simulink library "carnot"  (R2013b)
settings: Solver=ode45  StartTime=0.0  StopTime=10.0  RelTol=1e-3
undefined symbols (not defined in the file or in its folder): A, acol, Ahabit, Awin, Azimuth_Angle, AziWin, B, C, c1, c4, capc, caph, CarnotCallbacks_Density, CarnotCallbacks_Enthalpy, CarnotCallbacks_Enthalpy2Temperature, CarnotCallbacks_Entropy, CarnotCallbacks_Evaporation_Enthalpy, CarnotCallbacks_GlobalMessageLevel, CarnotCallbacks_Grashof, CarnotCallbacks_Heat_Capacity, CarnotCallbacks_Kinematic_Viscosity, CarnotCallbacks_Prandtl, CarnotCallbacks_Saturation_Property, CarnotCallbacks_Saturation_Temperature, CarnotCallbacks_Saturation_Value_Water, CarnotCallbacks_Specific_Volume, CarnotCallbacks_Thermal_Conductivity, CarnotCallbacks_Vapour_Content, CarnotCallbacks_Vapour_Pressure, con, cond, d, Dd, density, dfin, dia, DiameterLastPiece, DPConstant, dpipe, DPLinear, DPQuadratic, emission_out, fluid, FluidMix, FluidType, FPC, frame, g, GeodeticHeight, Gwin, heat_capacity, hgt, HP, Hroom, ID, inlet, K, l, lin, lpipe ... (+29)
undefined symbols (not defined in the file): c2, c3, c5, c6, cwall, dactive, height, mc, mID, rho, tau, UAneighbour, UAwall, uloss
libraries: carnot x333, simulink x25, simulink_extras x7
(part 1 of 16)
settings Model: Creator=awohlfei  LastModifiedBy=awohlfei

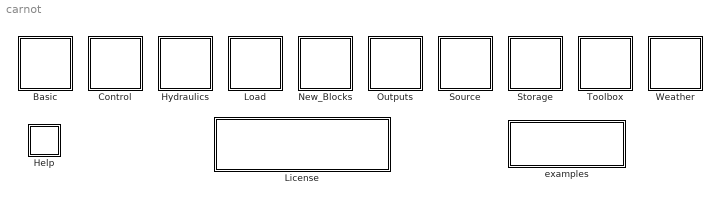
== system carnot ==
  Basic : Subsystem
      mask Display: plot(0,0,100,100,[10,10,40,40,10],[10,40,40,10,10],[50,70,90,50],[30,65,30,30],[20,10,10,20,30,40,40,30,20],[50,60,70,80,80,70,60,50,50])
  Control : Subsystem
      mask Display: plot(0,0,100,100,[70,100,40,10,70,70,10,10],[50,80,80,50,50,20,20,50],[100,70],[50,20],[20,50,50,20,20],[40,40,30,30,40],[62,62,62,61,59,58,58,60],[42,41,39,38,38,40,42,43],[61,62,62,61,60,59,58,58,58,59],[32,31,30,28,27,28,28,30,31,32])
  Help : Subsystem
      settings: OpenFcn=manual
      mask Display: disp('?');
  Hydraulics : Subsystem
      mask Display: plot(0,0,100,100,[15,18,18,15,40,40,46,55,60,60,55,46,40,40,15,10,10,15],[60,53,46,40,40,20,24,24,20,80,85,85,80,60,60,53,46,40],[60,55,46,40],[20,15,15,20])
  License : Subsystem
      mask Display: disp('Carnot 6.0\nfor MATLAB R2013b\nCopyright Solar-Institute Juelich');
  Load : Subsystem
      mask Display: plot(0,0,100,100,[10,20,30,10,30,30,10,10],[30,50,30,30,30,10,10,30],[30,20,10,30,30,10,10],[80,100,80,80,60,60,80],[77,76,70,50],[70,76,80,80],[74,66],[90,90],[70,70],[80,89],[77,76,70,50],[20,26,30,30],[74,66],[40,40],[70,70],[30,39])
  New_Blocks : Subsystem
      mask Display: plot(0,0,100,100,[80,20],[10,10],[70,55,45,30],[10,90,90,10])
  Outputs : Subsystem
      mask Display: plot(0,0,100,100,[90,10,10],[10,10,90],[90,80,70,60,50,10],[65,63,50,26,20,20],[90,70,57,46,40,31,40,50,60,70,90],[78,78,72,60,36,20,20,33,60,70,70],[90,60,45,31,24,21,14,21,30,34,44,59,90],[87,87,85,75,58,35,20,20,37,58,77,83,83])
  Source : Subsystem
      mask Display: plot(0,0,100,100,[30,40,60,70,70,30,30],[50,44,44,50,10,10,50],[50,50],[44,57],[50,46,44,46,50,54,56,54,50],[93,85,70,54,48,54,70,85,93])
  Storage : Subsystem
      mask Display: plot(10,10,90,100,[40,40,45,55,60,60,55,45,40],[84,36,30,30,36,84,90,90,84],[40,35],[77,77],[64,60],[77,77],[40,35],[42,42],[64,60],[42,42])
  Toolbox : Subsystem
      mask Display: plot(0,0,100,100,[10,40,50,40,10,10],[90,90,80,70,70,90],[28,28,22,22],[70,10,10,70],[70,80,80,70,70],[50,50,10,10,50],[77,77],[10,50],[73,73],[10,50],[76,76,74,74],[50,90,90,50])
  Weather : Subsystem
      mask Display: plot(7,7,95,100,[10,7,10,20,30,23,25,40,54,56,50,60,70,73,70,60,20,10],[15,24,34,40,35,42,50,55,50,42,35,40,34,24,15,10,10,15],[70,60,60,70,80,90,90,80,70],[90,80,70,60,60,70,80,90,90],[75,75],[91,97],[75,75],[52,58],[58,52],[75,75],[98,91],[75,75],[63,58],[63,57],[92,86],[92,87],[63,58],[85,92],[92,86],[57,64])
  examples : Subsystem
      settings: OpenFcn=|
      | filepath = '\public\tutorial\examples';
      | oldpath = pwd;
      | cd(fullfile(path_carnot('root'),filepath));
      | [filename, pathname, filterindex] = ...
      | uigetfile( { '*.mdl', ...
      | 'house examples'; ...
      | '*.mdl','MAT-files (*.mat)'; ...
      | '*.*',  'All Files (*.*)'},  'Pick an example');
      | if (filterindex > 0)
      |    open_system(fullfile(pathname,filename));
      | end
      | cd(oldpath);
      mask Display: disp('double click \nto load examples');

== system carnot/Basic ==
  Hydraulics : Subsystem
      mask Display: plot(0,0,100,100,[15,18,18,15,40,40,46,55,60,60,55,46,40,40,15,10,10,15],[60,53,46,40,40,20,24,24,20,80,85,85,80,60,60,53,46,40],[60,55,46,40],[20,15,15,20])
  Material_Properties : Subsystem
      mask Display: plot(10,10,80,80,[30,25,20,25,30,30,40,40,25,10,10,20,20],[60,59,60,61,60,50,32,30,27,30,32,50,60],[50,54,54,50,60,68,70,60,50,45,40,40,44,50],[60,64,70,72,70,67,70,75,77,77,73,65,60,60],[70,65,60,65,70,70,67,64,60],[50,51,50,48,50,15,10,10,15],[60,60],[15,50])
  Pressure_Drop : Subsystem
      mask Display: plot(0,0,100,100,[10,10,40,40,10],[10,40,40,10,10],[50,70,90,50],[30,65,30,30],[20,10,10,20,30,40,40,30,20],[50,60,70,80,80,70,60,50,50])
  Thermal_Models : Subsystem
      mask Display: plot(0,0,100,100,[10,10,40,40,10],[10,40,40,10,10],[50,70,90,50],[30,65,30,30],[20,10,10,20,30,40,40,30,20],[50,60,70,80,80,70,60,50,50])
  Ventilation : Subsystem
      mask Display: plot(0,0,100,100,[10,10,40,40,10],[10,40,40,10,10],[50,70,90,50],[30,65,30,30],[20,10,10,20,30,40,40,30,20],[50,60,70,80,80,70,60,50,50])
  Weather_and_Sun : Subsystem
      mask Display: plot(7,7,95,100,[10,7,10,20,30,23,25,40,54,56,50,60,70,73,70,60,20,10],[15,24,34,40,35,42,50,55,50,42,35,40,34,24,15,10,10,15],[70,60,60,70,80,90,90,80,70],[90,80,70,60,60,70,80,90,90],[75,75],[91,97],[75,75],[52,58],[58,52],[75,75],[98,91],[75,75],[63,58],[63,57],[92,86],[92,87],[63,58],[85,92],[92,86],[57,64])

== system carnot/Control ==
  Controller_Bang_Bang : Subsystem  mask(bang bang controler){deltaTon=5, deltaToff=1, Tmax=95}
      mask prompts: deltaTon "deltaT-on [K]"; deltaToff "deltaT-off [K]"; Tmax "maximum temperature [degree centigrade]"
      mask help:
      | Hysteresis controller for thermal systems. Output is set to zero if Thot or Tcold is bigger than Tmax.
      | deltaT = Thot - Tcold
      mask Help: web(fullfile(path_carnot('help'),'Controller_Bang_Bang.html'),'-helpbrowser')
      mask Display: plot(-30,0,150,100,[70,100,40,10,70,70,10,10],[50,80,80,50,50,20,20,50],[100,70],[50,20],[20,50,50,20,20],[40,40,30,30,40],[62,62,62,61,59,58,58,60],[42,41,39,38,38,40,42,43],[61,62,62,61,60,59,58,58,58,59],[32,31,30,28,27,28,28,30,31,32])
  EnergyMeter : Subsystem  mask(energy meter){}
      mask help: Calculates the power and energy of a fluid flow between inlet and outlet of components.
      mask Help: web(fullfile(path_carnot('help'),'EnergyMeter.html'),'-helpbrowser')
  EnergyMeter_HC : Subsystem  mask(energy meter Heating/Cooling){}
      mask help:
      | Calculates the power and energy of a fluid flow between inlet and outlet of components.
      | Positive power is integrated to the heating energy, negative power is integrated to the cooling energy.
      mask Help: eval('htmlhelp (''chap_4_2e.htm#energy_meter'')');
  Massflow_Sensor : Subsystem  mask(temperature measurement sensor){tc=10, t0=0}
      mask prompts: tc "time constant of sensor [s]"; t0 "initial value [kg/s]"
      mask help: Measurement sensor for temperatures with first-oder hold. Temperature is in degree centigrade.
      mask init:
      | tc = 1/max(tc, 0.001);
      mask Help: web(fullfile(path_carnot('help'),'Massflow_Sensor.html'),'-helpbrowser')
  Max_Run_Time : Subsystem  mask(Maximum Running Time){tmaxrun=5}
      mask prompts: tmaxrun "Maximum operation time in s"
      mask help: Keeps the output to the input level until either the maximum running time is reached or the input is set to zero.
      mask Help: web(fullfile(path_carnot('help'),'Max_Run_Time.html'),'-helpbrowser')
      mask Display:
      | plot(-20,-30,120,100,[10,20,40,60,80,90,90,80,60,40,20,10,10],[40,20,10,10,20,40,60,80,90,90,80,60,40],[55,46],[95,95],[50,50],[90,95],[50,50,24],[88,50,66],[10,13],[50,50],[90,87],[50,50],[50,50],[10,15])
      | disp('\n\nMax On')
  Min_Run_Time : Subsystem  mask(Minimum Running Time){tminrun=2, mv=2}
      mask prompts: tminrun "Minimum operation time in s"; mv "Minimum output value"
      mask help: Once started, the output is kept to the maximum of the input value and the mimimum output for at least the minimum running time.
      mask Help: web(fullfile(path_carnot('help'),'Min_Run_Time.html'),'-helpbrowser')
      mask Display:
      | plot(-20,-30,120,100,[10,20,40,60,80,90,90,80,60,40,20,10,10],[40,20,10,10,20,40,60,80,90,90,80,60,40],[55,46],[95,95],[50,50],[90,95],[50,50,24],[88,50,66],[10,13],[50,50],[90,87],[50,50],[50,50],[10,15])
      | disp('\n\nMin On')
  Min_Stop_Time : Subsystem  mask(Minimum Stop Time){tminstop=15}
      mask prompts: tminstop "Minimum stop time in s"
      mask help: Once stopped, the output is held to zero for at least the minimum stop time.
      mask Help: web(fullfile(path_carnot('help'),'Min_Stop_Time.html'),'-helpbrowser')
      mask Display:
      | plot(-20,-30,120,100,[10,20,40,60,80,90,90,80,60,40,20,10,10],[40,20,10,10,20,40,60,80,90,90,80,60,40],[55,46],[95,95],[50,50],[90,95],[50,50,24],[88,50,66],[10,13],[50,50],[90,87],[50,50],[50,50],[10,15])
      | disp('\n\nMin Off')
  OnOff_switch : Constant  Value=0
      settings: OpenFcn=set_param(gcb,'value',num2str(1-str2num(get_param(gcb,'value'))))
  PowerMeter : Subsystem  mask(power meter){}
      mask help:
      | Calculates the power of a fluid flow between inlet and outlet of components characterized by the THB.
      | Qdot = mdot * cp(Tmean) * (Tout - Tin)
      | Tmean = (Tin+Tout)/2
      mask Help: web(fullfile(path_carnot('help'),'PowerMeter.html'),'-helpbrowser')
  Solar_Radiation_Sensor : Subsystem  mask(measure solar radiation){rad=diffuse, rad_typ=normal to the beam radiation}
      mask prompts: rad "measured radiation"; rad_typ "orientation of the sensor"
      mask help:
      | Extracts the solar radiation in W/m² from the weather data vector.
      |
      | WARNING:
      | For old weather data vectors, their is only one type of tsolar radiation.
      mask init:
      | if (rad_typ == 1)
      |     if (rad == 1)
      |         vector = [3];
      |     elseif (rad == 2)
      |         vector = [4];
      |     else
      |         vector = [3 4];
      |     end
      | else
      |     if (rad == 1)
      |         vector = [16];
      |     elseif (rad == 2)
      |         vector = [17];
      |     else
      |         vector = [16 17];
      |     end
      | end
      mask Help: web(fullfile(path_carnot('help'),'Solar_Radiation_Sensor.html'),'-helpbrowser')
      mask TypeOptions rad: direct | diffuse | global
      mask TypeOptions rad_typ: normal to the beam radiation | fixed (horizontal or inclined)
  Start_Delay : Subsystem  mask(Start Delay){tstartdelay=5}
      mask prompts: tstartdelay "Start delay time in s"
      mask help: The output is delayed for the delay time, than it equal to the input.
      mask Help: web(fullfile(path_carnot('help'),'Start_Delay.html'),'-helpbrowser')
      mask Display:
      | plot(-20,-30,120,100,[10,20,40,60,80,90,90,80,60,40,20,10,10],[40,20,10,10,20,40,60,80,90,90,80,60,40],[55,46],[95,95],[50,50],[90,95],[50,50,24],[88,50,66],[10,13],[50,50],[90,87],[50,50],[50,50],[10,15])
      | disp('\n\nDelay On')
  T_Sensor : Subsystem  mask(temperature measurement sensor){tc=10, t0=20}
      mask prompts: tc "time constant of sensor [s]"; t0 "initial temperature [degree centigrade]"
      mask help: Measurement sensor for temperatures with first-oder hold. Temperature is in degree centigrade.
      mask init:
      | tc = 1/max(tc, 0.001);
      mask Help: web(fullfile(path_carnot('help'),'T_Sensor.html'),'-helpbrowser')
      mask Display: plot(0,0,100,100,[50,55,65,70,70,65,55,45,35,30,30,35,44,50,50],[50,50,60,70,80,90,100,100,90,80,70,60,50,50,-0],[60,40],[90,90],[50,50],[57,90])
  T_Sensor_Surface : Subsystem  mask(surface temperature sensor){pos=[0.1 0.4 0.5 0.9], tdel=1, t0=20}
      mask prompts: pos "relative position 0..1 (0 = bottom, 1 = top)"; tdel "delay-time in s"; t0 "initial temperature in degree centigrade"
      mask help:
      | Surface temperature sensor for a storage. The block breaks the algebraic loop when connecting the node temperature directly to the controller.
      | The relative position can be a vector for several sensors, for example [0.1 0.5 0.9]
      mask init:
      | tdel = max(tdel,0.01);
      | pos = max(0, min(pos, 1));
      mask Help: web(fullfile(path_carnot('help'),'T_Sensor_Surface.html'),'-helpbrowser')
      mask Display: plot(-10,0,110,100,[50,55,65,70,70,65,55,45,35,30,30,35,44,50,50],[50,50,60,70,80,90,100,100,90,80,70,60,50,50,-0],[60,40],[90,90],[50,50],[57,90])
  Window_Control : Subsystem  mask(Window Control){}
      mask help: Control for free driven passive cooling realized by tilted windows.
      mask Help: web(fullfile(path_carnot('help'),'Window_Control.html'),'-helpbrowser')

== system carnot/Help ==

== system carnot/Hydraulics ==
  Flow_Diverter : Subsystem  mask(flow diverter, fixed rate){}
      mask help:
      | The block diverts an incoming massflow according to:
      | mdot1 = mdot * fdiv
      | mdot2 = mdot * (1-fdiv)
      | fdiv is limited to the range [0..1]
      mask Help: web(fullfile(path_carnot('help'),'Flow_Diverter.html'),'-helpbrowser')
      mask Display: plot(0,-5,120,65,[20 45 20 20],[20 30 40 20],[45 70 70 45],[30 20 40 30],[45 35 55 45],[30 10 10 30])
  Flow_Mixer : Subsystem  mask(flow mixer){t=10}
      mask prompts: t "time constant of mixer"
      mask help: Mixes two massflows. The new temperature is calculated by an energy balance. The output f_div may be fed back to the corresponding flow diverter upwards in flowdirection.
      mask init:
      | if t < 0.0001
      |     t = 0.0001;
      |     disp('warning in Flow Mixer: Time constant set to 0.0001')
      | end
      mask Help: web(fullfile(path_carnot('help'),'Flow_Mixer.html'),'-helpbrowser')
      mask Display: plot(-25,-5,95,65,[20 45 20 20],[20 30 40 20],[45 70 70 45],[30 20 40 30],[45 35 55 45],[30 10 10 30])
  Flow_Mixer_Thermostatic : Subsystem  mask(thermostatic flow mixer){t=10}
      mask prompts: t "time constant for valve [s]"
      mask help:
      | The thermostatic flow mixer mixes cold and hot fluid to set a desired temperature and calculates the pressure drop.
      | Use together with flow_diverter_fixed_rate.
      mask init:
      | if t < 0.01
      |     t = 0.01;
      |     disp('Flow mixer thermostatic: time constant set to minimum value 0.01')
      | end
      | t1 = 1/t;
      mask Help: web(fullfile(path_carnot('help'),'Flow_Mixer.html'),'-helpbrowser')
      mask Display: plot(10,0,100,100,[40,60,60,40,40],[60,40,60,40,60],[44,50,56,44],[66,50,66,66],[50,50],[30,50],[56,44],[25,25],[50,50],[10,25])
  Pipe : Subsystem  mask(pipe){dia=0.02, len=10, hgt=5, uloss=100/20/10, cond=0, cwall=1000, t0=20, lin=100/0.2, qua=100/0.2^2, nodes=10}
      mask prompts: dia "diameter [m]"; len "length of pipe [m]"; hgt "static height [m], positive for outlet above"; uloss "heat losses per length [W/(m*K)]"; cond "effective conductivity in axial direction [W/(m*K)]"; cwall "capacity of pipewall per length in [J/(m*K)]"; t0 "initial temperature [degree Celsius]"; lin "pressure drop linear in massflow [Pa*s/kg]"; qua "pressure drop quadratic in massflow [Pa*s²/kg²]"; nodes "number of nodes"
      mask help:
      | Multinode pipe with capacity and simlified pressure drop calculation. The pressure drop is a quadratic function of the massflow. The dependance of the quadratic term on the Reynolds number is neglected. The flow is calculated by the upwind scheme heat conduction between nodes by central differences (Patankar 1980).
      | heat loss: ul = 2*Conductivity*pi*d_in*Length/Length/(d_in*ln(d_out/d_in))
      | The pressure change due to static height can usually be neglected for closes loop pumped systems.
      mask init:
      | if dia < 0.001
      |     dia = 0.001;
      |     disp('Warning in Pipe: diameter set to minimum value 0.001 m')
      | end
      | if len < 0.001
      |     len = 0.001;
      |     disp('Warning in Pipe: length set to minimum value 0.001 m')
      | end
      | if cwall < 0.001
      |     cwall = 0.001;
      |     disp('Warning in Pipe: heat capacity of the wall set to minimum value 0.001 m')
      | end
      | if nodes < 1
      |     nodes = 1;
      |     disp('Warning in Pipe: number of nodes set to minimum 1')
      | end
      mask Help: web(fullfile(path_carnot('help'),'Pipe.html'),'-helpbrowser')
      mask Display: plot(0,0,100,100,[24,27,27,24,75,80,80,75,24,20,20,24],[60,53,46,40,40,46,55,60,60,53,46,40])
  Pipe_Geometry : Subsystem  mask(Pipe Geometry){dia=0.02, len=10, hgt=10, uloss=100/20/10, cond=0, cwall=1000, t0=20, rough=0.04*1e-3, nbend=4, nodes=1}
      mask prompts: dia "diameter [m]"; len "length of pipe [m]"; hgt "static height [m], (positive for outlet above inlet)"; uloss "heat loss per length of pipe [W/(m*K)]"; cond "effective conductivity in the pipe [W/(m*K)]"; cwall "capacity of pipewall per length [J/(m*K)]"; t0 "initial temperature [degree centigrade]"; rough "roughness of pipe [m]"; nbend "number of 90° bends (45° = 0.667)"; nodes "number of nodes"
      mask help:
      | Multinode pipe with capacity and theoretical pressure drop calculation. The flow is calculated by the upwind scheme heat conduction between nodes by central differences (Patankar 1980).
      | heat loss: ul = 2*Conductivity*pi*d_in*Length/Length/(d_in*ln(d_out/d_in))
      | The pressure change due to static height can usually be neglected for closes loop pumped systems.
      mask init:
      | if dia < 0.001
      |     dia = 0.001;
      |     disp('Warning in Pipe: diameter set to minimum value 0.001 m')
      | end
      | if len < 0.001
      |     len = 0.001;
      |     disp('Warning in Pipe: length set to minimum value 0.001 m')
      | end
      | if cwall < 0.001
      |     cwall = 0.001;
      |     disp('Warning in Pipe: heat capacity of the wall set to minimum value 0.001 m')
      | end
      | if nodes < 1
      |     nodes = 1;
      |     disp('Warning in Pipe: number of nodes set to minimum 1')
      | end
      | if nbend < 0
      |     nbend = 0;
      |     disp('Warning in Pipe: number of bends set to minimum 0')
      | end
      | if rough < 0
      |     rough = 0;
      |     disp('Warning in Pipe: roughness of nodes set to minimum 0 m')
      | end
      mask Help: web(fullfile(path_carnot('help'),'Pipe_Geometry.html'),'-helpbrowser')
      mask Display: plot(0,0,90,100,[8,12,16,16,12,8,8],[46,38,46,55,62,55,46],[12,33,48,52,70,73,73,70,50,35,30,12],[38,49,30,30,50,55,65,70,50,70,70,62])
  Pipe_Isolation : Subsystem  mask(pipe with relative isolation thickness){dia=0.02, len=10, hgt=0, isolat=43.72, condiso=0.05, cond=0, cwall=1000, t0=20, lin=100/0.2, qua=100/0.2^2, nodes=10}
      mask prompts: dia "Diameter [m]"; len "Length of pipe [m]"; hgt "difference in static height [m], positive for outlet above"; isolat "Isolation thickness in % (100%: isolation thickness = diameter, minimum 1%)"; condiso "Thermal conductivity of isolation [W/(m*K)]"; cond "Effective conductivity in the pipe [W/(m*K)]"; cwall "capacity of pipewall per length in [J/(m*K)]"; t0 "initial temperature [degree centigrade]"; lin "pressure drop linear in massflow [Pa*s/kg]"; qua "pressure drop quadratic in massflow [Pa*s²/kg²]"; nodes "number of nodes"
      mask help:
      | Multinode pipe with capacity and easy pressure drop calculation. The pressure drop is a quadratic function of the massflow. The dependance of the quadratic term on the Reynolds number is neglected. The flow is calculated by the upwind scheme heat conduction between nodes by central differences (Patankar 1980).
      | Isolation thickness in percent of the diameter. Heat loss:
      | ul = 2*conductivity*pi*d*Length/Length/(d*log(((2*percent+1)d)/d))
      | The pressure change due to static height can usually be neglected for closes loop pumped systems.
      mask init:
      | if dia < 0.001
      |     dia = 0.001;
      |     disp('Warning in Pipe: diameter set to minimum value 0.001 m')
      | end
      | if len < 0.001
      |     len = 0.001;
      |     disp('Warning in Pipe: length set to minimum value 0.001 m')
      | end
      | if cwall < 0.001
      |     cwall = 0.001;
      |     disp('Warning in Pipe: heat capacity of the wall set to minimum value 0.001 m')
      | end
      | if nodes < 1
      |     nodes = 1;
      |     disp('Warning in Pipe: number of nodes set to minimum 1')
      | end
      | if isolat < 1
      |     isolat = 1;
      |     disp('Warning in Pipe: Isolation set to minimum 1%')
      | end
      | uloss = 2*condiso*pi/(log(0.01*isolat*2+1));
      mask Help: web(fullfile(path_carnot('help'),'Pipe_Isolation.html'),'-helpbrowser')
      mask Display: plot(-20,10,130,90,[0,2,5,7,5,2,0],[55,50,50,55,60,60,55],[96,99,100,99,96],[50,50,55,60,60],[10,13,17,19,19,17,13,10],[50,45,45,50,60,65,65,60],[5,15,17,17,15,5],[50,50,52,58,60,60],[17,93,96,96,92,17],[45,45,46,62,65,65])
  Pump_Additional : Subsystem  mask(additional pump){a0=2.0e4, a1=-7000, a2=0 %-3e-3, dia=0.025, t1=5, ua=0, mcp=0, tamb=0}
      mask prompts: a0 "pump characteristic: constant coefficient [Pa]"; a1 "pump characteristic: linear coefficient [Pa*s/kg]"; a2 "pump characteristic: quadratic coefficient [Pa*(s/kg)²]"; dia "diameter at in- and outlet [m]"; t1 "time constant in s"; ua "losses to ambient  in W/K"; mcp "thermal capacity in J/K"; tamb "ambient temperatature in °C"
      mask help: This pump is an additional pump in a circuit. Every circuit must have exactly ONE 'pump_main'. It may have several 'pump_additional' blocks.
      mask init:
      | t=1;
      mask Help: web(fullfile(path_carnot('help'),'Pump_Main.html'),'-helpbrowser')
      mask Display:
      | plot(0,0,100,100,[40,70,40,30,30,40,60,70,70,60,40],[70,50,30,40,60,70,70,60,40,30,30])
      | port_label('input',1,'THB')
      | port_label('input',2,'ctr')
      | port_label('output',1,'THB')
      | port_label('output',2,'Pel')
  Pump_Const : Subsystem  mask(constant pump){mdotmax=1200/3600, dia=0.0157, power=30, p0=3e5, fluid_id=Water, mix=0, UA=3, mcp=4000, tamb=20}
      mask prompts: mdotmax "massflow rate [kg/s]"; dia "diameter at in- and outlet [m]"; power "electric power consumption [W]"; p0 "system pressure in Pa"; fluid_id "fluid"; mix "percentage of fluid mix [0..1]"; UA "losses to ambient in W/K"; mcp "thermal capacity in J/K"; tamb "ambient temperatature in °C"
      mask help:
      | Set constant massflow rate according to the control signal.
      | The pump has a thermal capacity and losses to ambient.
      mask Help: web(fullfile(path_carnot('help'),'Pump_Const.html'),'-helpbrowser')
      mask TypeOptions fluid_id: Water | Air | Cotton Oil | Silicone Oil | Water-Glycol Mix | Tyfocor LS | Water (Constant 20°C) | Air (dry+ constant 20°C)
      mask Display:
      | plot(0,0,100,100,[40,70,40,30,30,40,60,70,70,60,40],[70,50,30,40,60,70,70,60,40,30,30])
      | port_label('input',1,'THB')
      | port_label('input',2,'ctr')
      | port_label('output',1,'THB')
      | port_label('output',2,'Pel')
  Pump_Main : Subsystem  mask(main pump){a0=2.7e4, a1=-1.2e4, a2=-3e-3, dia=0.025, t1=5, p0=3e5, IDchk=off, fluid_id=Water, mix=0, ua=1, mcp=500, tamb=20}
      mask prompts: a0 "constant coefficient a0 [Pa]"; a1 "linear coefficient a1 [Pa*s/kg]"; a2 "quadratic coefficient a2 [Pa*(s/kg)²]"; dia "diameter at in- and outlet [m]"; t1 "time constant in s"; p0 "system pressure in Pa"; IDchk "calculate static pressure in system"; fluid_id "fluid"; mix "percentage of fluid mix [0..1]"; ua "losses to ambient  in W/K"; mcp "thermal capacity in J/K"; tamb "ambient temperatature in °C"
      mask help:
      | This is the main pump in a circuit. Every circuit must have exactly ONE 'Pump_Main'. Use the 'pump_additional' blocks if you want to use more pumps.
      | Calculate massflow by solving the equations:
      |     pressure_drop = c + l*mdot + q*(mdot)²
      |     pump_pressure = a0 + a1*mdot +a2*(mdot)²
      |     with: pressure_drop = pump_pressure
      | The system pressure specified as parameter is the pressure at the outlet of the pump. All pressure drops in the circuit will reduce this pressure.
      mask init:
      | ID = IDchk*10000+10001;
      mask Help: web(fullfile(path_carnot('help'),'Pump_Main.html'),'-helpbrowser')
      mask TypeOptions fluid_id: Water | Air | Cotton Oil | Silicone Oil | Water-Glycol Mix | Tyfocor LS | Water (Constant 20°C) | Air (dry+ constant 20°C)
      mask Display:
      | plot(0,0,100,100,[40,70,40,30,30,40,60,70,70,60,40],[70,50,30,40,60,70,70,60,40,30,30])
      | port_label('input',1,'THB')
      | port_label('input',2,'ctr')
      | port_label('output',1,'THB')
      | port_label('output',2,'Pel')
  Pump_Simple : Subsystem  mask(simple Pump){mdotmax=1200/3600, dia=0.0157, power=30, fluid_id=Water, mix=0, p0=3e5}
      mask prompts: mdotmax "massflow rate [kg/s]"; dia "diameter at in- and outlet [m]"; power "electric power consumption [W]"; fluid_id "fluid"; mix "percentage of fluid mix [0..1]"; p0 "system pressure [Pa]"
      mask help:
      | Set constant massflow rate according to the control signal.
      | The pump is a very basic model, sometimes creating algebraic loops. If you have problems with algebraic loops, use "Pump_const" instead.
      mask Help: web(fullfile(path_carnot('help'),'Pump_Const.html'),'-helpbrowser')
      mask TypeOptions fluid_id: Water | Air | Cotton Oil | Silicone Oil | Water-Glycol Mix | Tyfocor LS | Water (Constant 20°C) | Air (dry+ constant 20°C)
      mask Display:
      | plot(0,0,100,100,[40,70,40,30,30,40,60,70,70,60,40],[70,50,30,40,60,70,70,60,40,30,30])
      | port_label('input',1,'THB')
      | port_label('input',2,'ctr')
      | port_label('output',1,'THB')
      | port_label('output',2,'Pel')
  Thermosyphon : Subsystem  mask(thermosyphon){dia=0.025, fluid_id=water, mix=0, p0=2e5, t1=5}
      mask prompts: dia "diameter at in- and outlet [m]"; fluid_id "fluid"; mix "percentage of fluid mix [0..1]"; p0 "system pressure in [Pa]"; t1 "time constant in s"
      mask help:
      | This block is a model of a "thermosyphon pump". Place it in natural convection systems as you would place a pump.
      | Assure that the sum of heights is zero. Otherwise the simulation will not start.
      | You may check the sum of heights by verifying the "Geodetic Height" in the THB at the inport of this block.
      | If the sum is not zero, the difference is displayed in the subsystem "Stop Simulation".
      mask Help: web(fullfile(path_carnot('help'),'Thermosyphon.html'),'-helpbrowser')
      mask TypeOptions fluid_id: water | air | cotton oil | silicone oil | water-glycol mix | Tyfocor LS
      mask Display:
      | plot(0,0,100,100,[90,10],[80,90],[90,10],[70,80],[90,10],[20,10],[90,10],[30,20],[40,60,40,40],[60,50,40,60])
      | port_label('input',1,'THB')
      | port_label('output',1,'THB')
  Valve : Subsystem  mask(valve){pos_values=[0 0.1 1], dp_values=[1e6 1e6 1]}
      mask prompts: pos_values "position (vector with values 0..1)"; dp_values "QUA : quadratic pressure drop (vector)"
      mask help:
      | The block calculates the pressure drop at a valve. The characteristic is defined by a lookup table for QUA:
      | dp = QUA * mdot^2
      mask Help: web(fullfile(path_carnot('help'),'Valve.html'),'-helpbrowser')
      mask Display: plot(-15,0,115,100,[30,70,70,30,30],[60,40,60,40,60],[60,40],[80,80],[50,50],[50,80])
  Valve_ThermoTset : Subsystem  mask(thermostatic valve){p=3, op=0.5, bl=10, ts=30, dia=0.02, vpos=[0 0.1 1], vqua=[1e6 1e6 1]}
      mask prompts: p "proportional Range [K]"; op "operating point [0..1] (valve position at set temperature)"; bl "play hysteresis []"; ts "first-order hold ts [s]"; dia "diameter [m]"; vpos "Valve position vector [0..1]"; vqua "Vector with quadratic pressure drop in massflow in Pa*s²/kg²"
      mask help:
      | Thermostatic valve for a radiator.
      | set temperature and slope
      | valve position = -slope * (T(sensor) - Toffset)
      mask init:
      | % p=1/p;
      | % op = min(1, max(0, op));
      | % tu = max(tu,0);
      | % ts = max(ts,0);
      | % dia = max(dia, 0.001);
      | %
      mask Help: web(fullfile(path_carnot('help'),'Valve_Thermostatic.html'),'-helpbrowser')
      mask Display:
      | plot(-30,-10,130,110,[20,80,80,20,20],[60,30,60,30,60],[50,50],[45,70],[60,40],[96,96],[50,50],[75,96])
      | port_label('input',1,'THB')
      | port_label('input',2,'Troom')
      | port_label('input',3,'Tset')
      | port_label('output',1,'THB')
  Valve_ThermoTset_fn : Subsystem  mask(thermostatic valve with Kv function){p=3, op=0.5, bl=0.1, ts=30, dia=0.02, kv=0.6, kvs=0.8}
      mask prompts: p "proportional Range [K]"; op "operating point [0..1] (valve position at set temperature)"; bl "play hysteresis [K]"; ts "first-order hold ts [s]"; dia "diameter [m]"; kv "kv value"; kvs "kvs value"
      mask help:
      | Thermostatic valve for a radiator.
      | set temperature and slope
      | valve position = -slope * (T(sensor) - Toffset)
      mask Help: web(fullfile(path_carnot('help'),'Valve_Thermostatic.html'),'-helpbrowser')
      mask Display:
      | plot(-30,-10,130,110,[20,80,80,20,20],[60,30,60,30,60],[50,50],[45,70],[60,40],[96,96],[50,50],[75,96])
      | % port_label('input',1,'THB')
      | % port_label('input',2,'Troom')
      | % port_label('input',3,'Tset')
      | % port_label('output',1,'THB')
  Valve_Thermostatic : Subsystem  mask(thermostatic valve){Tset=20, prange=3, op=0.5, bl=0.1, ts=30, dia=0.02, vpos=[0 0.1 1], vqua=[1e6 1e6 1]}
      mask prompts: Tset "set temperature [degree centigrade]"; prange "proportional Range [K]"; op "operating point [0..1] (valve position at set temperature)"; bl "play hysterersis in K"; ts "first-order hold ts [s]"; dia "diameter [m]"; vpos "Valve position vector [0..1]"; vqua "Vector with quadratic pressure drop in massflow in Pa*s²/kg²"
      mask help:
      | Thermostatic valve for a radiator.
      | set temperature and slope
      | valve position = -slope * (T(sensor) - Toffset)
      mask Help: web(fullfile(path_carnot('help'),'Valve_Thermostatic.html'),'-helpbrowser')
      mask Display:
      | plot(-20,-10,130,110,[20,80,80,20,20],[60,30,60,30,60],[50,50],[45,70],[60,40],[96,96],[50,50],[75,96])
      | port_label('input',1,'THB')
      | port_label('input',2,'Troom')
      | port_label('output',1,'THB')
  Valve_fn : Subsystem  mask(valve with Kv function){kv=0.7, kvs=0.9, op=0.5}
      mask prompts: kv "Kv value"; kvs "Kvs value"; op "Operation point [0..1]"
      mask help:
      | The block calculates the pressure drop at a valve. The characteristic is defined the function:
      | QUA = 2.8e6*(kv/(kvs*(2/(1+exp(-2/op*u(1)))-1)))^2
      | dp = QUA * mdot^2
      mask Help: web(fullfile(path_carnot('help'),'Valve_fn.html'),'-helpbrowser')
      mask Display: plot(-15,0,115,100,[30,70,70,30,30],[60,40,60,40,60],[60,40],[80,80],[50,50],[50,80])

== system carnot/License ==
  note: This file is part of the CARNOT Blockset.
      | 	Copyright (c) 1998-2015, Solar-Institute Juelich of the FH Aachen.
      | 	Additional Copyright for file and models see list auf authors.
      | 	All rights reserved.
      | 	Redistribution and use in source and binary forms, with or without
      | 	modification, are permitted provided that the following conditions are met:
      | 	1. Redistributions of source code must retain the above copyright notice,
      | 	   this list of conditions and the following disclaimer.
      | 	2. Redistributions in binary form must reproduce the above copyright
      | 	   notice, this list of conditions and the following disclaimer in the
      | 	   documentation and/or other materials provided with the distribution.
      | 	3. Neither the name of the copyright holder nor the names of its
      |
      |    contributors may be used to endorse or promote products derived from
      |    this software without specific prior written permission.
      | THIS SOFTWARE IS PROVIDED BY THE COPYRIGHT HOLDERS AND CONTRIBUTORS "AS IS"
      | 	AND ANY EXPRESS OR IMPLIED WARRANTIES, INCLUDING, BUT NOT LIMITED TO, THE
      | 	IMPLIED WARRANTIES OF MERCHANTABILITY AND FITNESS FOR A PARTICULAR PURPOSE
      | 	ARE DISCLAIMED. IN NO EVENT SHALL THE COPYRIGHT HOLDER OR CONTRIBUTORS BE
      | 	LIABLE FOR ANY DIRECT, INDIRECT, INCIDENTAL, SPECIAL, EXEMPLARY, OR
      | 	CONSEQUENTIAL DAMAGES (INCLUDING, BUT NOT LIMITED TO, PROCUREMENT OF
      | 	SUBSTITUTE GOODS OR SERVICES; LOSS OF USE, DATA, OR PROFITS; OR BUSINESS
      | 	INTERRUPTION) HOWEVER CAUSED AND ON ANY THEORY OF LIABILITY, WHETHER IN
      | 	CONTRACT, STRICT LIABILITY, OR TORT (INCLUDING NEGLIGENCE OR OTHERWISE)
      | 	ARISING IN ANY WAY OUT OF THE USE OF THIS SOFTWARE, EVEN IF ADVISED OF
      | 	THE POSSIBILITY OF SUCH DAMAGE.

== system carnot/Load ==
  General : Subsystem
      mask Display: plot(0,0,100,100,[100,0,0],[-0,-0,100],[100,95,81,72,62,54,51,36,26,20,17,15,13,10,0],[10,46,32,57,96,96,31,39,5,1,87,33,47,50,10])
  Hot_Water_Tapping : Subsystem
      mask Display: plot(0,0,100,100,[44,67,67,45,45,40,40,44],[80,80,72,72,60,60,76,80],[60,45],[90,90],[53,53],[80,90],[24,29,70,75,24],[30,10,10,30,30],[42,42],[32,58],[46,44],[34,54],[38,40],[34,56])
  Houses : Subsystem
      mask Display: plot(0,0,80,90,[30,30,60,60,30],[20,50,50,20,20],[47,47,56,56,47],[40,30,30,40,40],[42,42,34,34],[20,40,40,20],[62,45,28],[48,70,48])

== system carnot/New_Blocks ==
  ReadFile : Subsystem  mask(readfile){number=5, timedep=off, filename='invar.dat'}
      mask prompts: number "Number of columns (without time column) / variables"; timedep "depending on time"
      mask help:
      | This function reads a matrix or variables from a file.
      |
      | timedependend
      | A matrix is read with the given number of column, where the first value is the time variable. This time is compared to the simulation time, so data, which are not in the matrix, will be linear interpolated.
      | Comment lines have to begin with % or //.
      | When the simulation time exceeds the time in the file, the function reads the file from the beginning.
      |
      |
      | not timedependend
      | All variables (not a matrix) in the file are read in the first function call. Then at every call the same variables will be put out.
      |
      | OUTPUT VECTOR
      | matrix row, when timedependend, without time
      | all variables, when not timedependend
      mask Help: web(fullfile(path_carnot('help'),'ReadFile.html'),'-helpbrowser')
  ground_storage_U_tube : Subsystem  InitFcn=disp('ATTENTION: MODEL ground_storage_U-tube IS NOT VALIDATED !')  mask(borehole ground storage){ds=1, hs=1, dh=0.05, hh=1, ground=clay (humid), borehole=clay (humid), dp=0.02, kp=0.001, t0=10, rn=6, zn=6, mpts=3}
      mask prompts: ds "diameter of storage region [m]"; hs "depth of storage region [m]"; dh "diameter of borehole [m]"; hh "depth of borehole [m]"; borehole "borehole filling"; dp "diameter of pipe [m]"; kp "roughness of pipe [m]"; t0 "initial temperature [degree centigrade]"; rn "number of radial nodes"; zn "number of axial nodes"; mpts "number of measurement points"
      mask help:
      | Model for the calculation of an U-tube ground storage.
      | Look under mask to change the surface model.
      |
      | ATTENTION: MODEL IS NOT VALIDATED !
      mask init:
      | ds = max(ds, 0.001);
      | hs = max(hs, 0.001);
      | dh = max(dh, 0.001);
      | hh = min(hs, max(hh, 0.001));
      | cond=[0.7 1.88 1.45 2.9 0.58];
      | le = cond(ground);
      | cap = [1382400 1798200 2410560 2864160 1798200];
      | ce = cap(ground);
      | lh = cond(borehole);
      | ch = cap(borehole);
      mask Help: web(fullfile(path_carnot('help'),'ground_storage_U_tube.html'),'-helpbrowser')
      mask TypeOptions ground: sand (dry) | sand (saturated with water) | clay (humid) | clay (saturated with water)
      mask TypeOptions borehole: sand (dry) | sand (saturated with water) | clay (humid) | clay (saturated with water) | bentonit (83% water)
      mask Display: plot(0,10,100,90,[70,30],[80,80],[35,35,43,43,47,52,57,57,66,66,60,60,54,46,40,40,35],[84,87,87,20,13,13,21,87,87,84,84,20,10,10,20,84,84])

== system carnot/Outputs ==
  AIV_selector : Subsystem  mask(AIV DATA){e1=on, e2=off, e3=off, e4=off, e5=off, e6=off, e7=off, e8=off, e9=off}
      mask prompts: e1 "Ts          : sensitive temperature, °C"; e2 "Tc          : convective/air temperature, °C"; e3 "Tr           : radiative temperature, °C"; e4 "x_H2O   : absolute water mass in air, kg/kg air"; e5 "x_CO2   : absolute CO2 mass in air, kg/kg air"; e6 "rho         : density of air, kg/m^3"; e7 "cp          : specific heat capacity of air, J/(kg*K)"; e8 "p            : absolute air pressure, N/m^2"; e9 "nair_out : air volume change indoors-outdoors, 1/h"
      mask help:
      | This block delivers a user specified vector with elements of the [AIV] vector.
      |
      | [AIV] : vector from NODE block
      | [AIV]s : output vector with user selected elements from [AIV]
      |
      | The sequence of elements in the output vector is identical to the sequence of selected check boxes counted from to the top to the bottom.
      mask init:
      | % concatenate elements of output "v":
      | v = [];
      | if (e1==1) v = [v 1]; end
      | if (e2==1) v = [v 2]; end
      | if (e3==1) v = [v 3]; end
      | if (e4==1) v = [v 4]; end
      | if (e5==1) v = [v 5]; end
      | if (e6==1) v = [v 6]; end
      | if (e7==1) v = [v 7]; end
      | if (e8==1) v = [v 8]; end
      | if (e9==1) v = [v 9]; end
      mask Help: web(fullfile(path_carnot('help'),'AIV_selector.html'),'-helpbrowser')
      mask Display:
      | plot ([0.8 0.9], [0.32 0.32])
      | plot ([0.8 0.85], [0.32 0.1])
      | plot ([0.9 0.85], [0.32 0.1])
      | plot ([0.827 0.827], [0 0.05])
      | plot ([0.827 0.87], [0.05 0.05])
      | plot ([0.87 0.87], [0 0.05])
      | plot ([0.827 0.87], [0 0])
  Display_THB1 : Subsystem  mask(display THB){t=on, m=off, p=off, id=off, mix=off, d=off}
      mask prompts: t "temperature [degree centigrade]"; m "massflow [kg/s]"; p "pressure [Pa]"; id "fluid ID (1 = water, 2 = air, 3 = cotton oil, 4 = water-glycol)"; mix "fluid mix"; d "diameter [m]"
      mask help: Displays the ticked values from one THB.
      mask init:
      | v=[];
      | if (t)
      |     v  = [2];
      | end
      | if (m)
      |     v= [v 3];
      | end
      | if (p)
      |     v = [v 4];
      | end
      | if (id)
      |     v = [v 5];
      | end
      | if (mix)
      |     v = [v 6];
      | end
      | if (d)
      |     v = [v 7];
      | end
      mask Help: web(fullfile(path_carnot('help'),'display_THB.html'),'-helpbrowser')
  Display_THB2 : Subsystem  mask(display THB){t=on, m=off, p=off, id=off, mix=off, d=off}
      mask prompts: t "temperature [degree centigrade]"; m "massflow [kg/s]"; p "pressure [Pa]"; id "fluid ID (1 = water, 2 = air, 3 = cotton oil, 4 = water-glycol)"; mix "fluid mix"; d "diameter [m]"
      mask help: Displays the ticked values from two THB.
      mask init:
      | v=[];
      | if (t)
      |     v  = [2];
      | end
      | if (m)
      |     v= [v 3];
      | end
      | if (p)
      |     v = [v 4];
      | end
      | if (id)
      |     v = [v 5];
      | end
      | if (mix)
      |     v = [v 6];
      | end
      | if (d)
      |     v = [v 7];
      | end
      mask Help: web(fullfile(path_carnot('help'),'display_THB.html'),'-helpbrowser')
  Display_THB3 : Subsystem  mask(display THB){t=on, m=off, p=off, id=off, mix=off, d=off}
      mask prompts: t "temperature [degree centigrade]"; m "massflow [kg/s]"; p "pressure [Pa]"; id "fluid ID (1 = water, 2 = air, 3 = cotton oil, 4 = water-glycol)"; mix "fluid mix"; d "diameter [m]"
      mask help: Displays the ticked values from four THB.
      mask init:
      | v=[];
      | if (t)
      |     v  = [2];
      | end
      | if (m)
      |     v= [v 3];
      | end
      | if (p)
      |     v = [v 4];
      | end
      | if (id)
      |     v = [v 5];
      | end
      | if (mix)
      |     v = [v 6];
      | end
      | if (d)
      |     v = [v 7];
      | end
      mask Help: web(fullfile(path_carnot('help'),'display_THB.html'),'-helpbrowser')
  Display_THB4 : Subsystem  mask(display THB){t=on, m=off, p=off, id=off, mix=off, d=off}
      mask prompts: t "temperature [degree centigrade]"; m "massflow [kg/s]"; p "pressure [Pa]"; id "fluid ID (1 = water, 2 = air, 3 = cotton oil, 4 = water-glycol)"; mix "fluid mix"; d "diameter [m]"
      mask help: Displays the ticked values from four THB
      mask init:
      | v=[];
      | if (t)
      |     v  = [2];
      | end
      | if (m)
      |     v= [v 3];
      | end
      | if (p)
      |     v = [v 4];
      | end
      | if (id)
      |     v = [v 5];
      | end
      | if (mix)
      |     v = [v 6];
      | end
      | if (d)
      |     v = [v 7];
      | end
      mask Help: web(fullfile(path_carnot('help'),'display_THB.html'),'-helpbrowser')
  Display_THB5 : Subsystem  mask(display THB){t=on, m=off, p=off, id=off, mix=off, d=off}
      mask prompts: t "temperature  [degree centigrade]"; m "massflow [kg/s]"; p "pressure [Pa]"; id "fluid ID (1 = water, 2 = air, 3 = cotton oil, 4 = water-glycol)"; mix "fluid mix"; d "diameter [m]"
      mask help: Displays the ticked values from six THB.
      mask init:
      | v=[];
      | if (t)
      |     v  = [2];
      | end
      | if (m)
      |     v= [v 3];
      | end
      | if (p)
      |     v = [v 4];
      | end
      | if (id)
      |     v = [v 5];
      | end
      | if (mix)
      |     v = [v 6];
      | end
      | if (d)
      |     v = [v 7];
      | end
      mask Help: web(fullfile(path_carnot('help'),'display_THB.html'),'-helpbrowser')
  Display_THB6 : Subsystem  mask(display THB){t=on, m=off, p=off, id=off, mix=off, d=off}
      mask prompts: t "temperature  [degree centigrade]"; m "massflow [kg/s]"; p "pressure [Pa]"; id "fluid ID (1 = water, 2 = air, 3 = cotton oil, 4 = water-glycol)"; mix "fluid mix"; d "diameter [m]"
      mask help: Displays the ticked values from six THB.
      mask init:
      | v=[];
      | if (t)
      |     v  = [2];
      | end
      | if (m)
      |     v= [v 3];
      | end
      | if (p)
      |     v = [v 4];
      | end
      | if (id)
      |     v = [v 5];
      | end
      | if (mix)
      |     v = [v 6];
      | end
      | if (d)
      |     v = [v 7];
      | end
      mask Help: web(fullfile(path_carnot('help'),'display_THB.html'),'-helpbrowser')
  S_selector : Subsystem  mask(S_Selector){e1=on, e2=off, e3=off, e4=off, e5=off, e6=off, e7=off, e8=off, e9=off, e10=off, e11=off, e12=off, e13=off}
      mask prompts: e1 "Qdot_sol       : solar radition load, W"; e2 "Qdot_equip   : electric equipment load, W"; e3 "Qdot_light     : electric light load, W"; e4 "Qdot_pers     : person load, W"; e5 "Qdot_heat     : heating / cooling, W"; e6 "Qdot_air        : heating/cooling power of air change, W"; e7 "Qdot_c          : heat flow to convective node, W"; e8 "Qdot_r           : heat flow to radiative node, W"; e9 "mdot_air        : air mass flow, kg/s"; e10 "mdot_H2O    : water mass flow, kg/s"; e11 "mdot_CO2    : CO2 mass flow, kg/s"; e12 "Vdot_out2in  : air volume flow outdoors -> indoors, m^3/s"; e13 "Vdot_in2out  : air volume flow indoors -> outdoors, m^3/s"
      mask help:
      | This block delivers a user specified vector with elements of the [S] vector.
      |
      | [S] : vector from SOURCE or SINK block
      | [S]s : output vector with user selected elements from [S]
      |
      | The sequence of elements in the output vector is identical to the sequence of selected check boxes counted from to the top to the bottom.
      mask init:
      | % concatenate elements of output "v":
      | v = [];
      | if (e1==1) v = [v 1]; end
      | if (e2==1) v = [v 2]; end
      | if (e3==1) v = [v 3]; end
      | if (e4==1) v = [v 4]; end
      | if (e5==1) v = [v 5]; end
      | if (e6==1) v = [v 6]; end
      | if (e7==1) v = [v 7]; end
      | if (e8==1) v = [v 8]; end
      | if (e9==1) v = [v 9]; end
      | if (e10==1) v = [v 10]; end
      | if (e11==1) v = [v 11]; end
      | if (e12==1) v = [v 12]; end
      | if (e13==1) v = [v 13]; end
      mask Help: web(fullfile(path_carnot('help'),'S_selector.html'),'-helpbrowser')
      mask Display:
      | plot ([0.8 0.9], [0.32 0.32])
      | plot ([0.8 0.85], [0.32 0.1])
      | plot ([0.9 0.85], [0.32 0.1])
      | plot ([0.827 0.827], [0 0.05])
      | plot ([0.827 0.87], [0.05 0.05])
      | plot ([0.87 0.87], [0 0.05])
      | plot ([0.827 0.87], [0 0])
  Sensitive_Room_Temperature : Subsystem  mask(SENSITIVE TEMPERATURE){share_c=47}
      mask prompts: share_c "SHARE of convective sensitivity, [0,100%]:"
      mask help:
      | This block merges the convective and radiative zone node temperature to the SENSITIVE ZONE TEMPERATURE (weighted arithmetic average of both components).
      | [T] = [Tc; Tr]:  temperature vector of node, °C
      | Ts:              sensitive zone temperature, °C
      mask init:
      | blockname = gcb;
      | 
      | if (length(share_c)~=1) error(['PARAMETERS block "' blockname ': "SHARE of ..." must have only 1 entry !']); end;
      | if (share_c<0) | (share_c>100) error(['PARAMETERS block "' blockname '" : "SHARE of ..." must be within [0, 100%] !']); end;
      | share_c = share_c/100;
      mask Help: web(fullfile(path_carnot('help'),'Sensitive_room_temperature.html'),'-helpbrowser')
  THV_select : Subsystem  mask(select from THV){f=off, t=on, m=off, p=off, id=off, mix=off, d=off, dpcon=off, dplin=off, dpqua=off}
      mask prompts: f "flow identifier"; t "temperature [degree centigrade]"; m "massflow [kg/s]"; p "pressure [Pa]"; id "fluid ID (1 = water, 2 = air, 3 = cotton oil, 4 = water-glycol)"; mix "fluid mix"; d "diameter [m]"; dpcon "constant press. drop"; dplin "linear pressure drop"; dpqua "quadratic pressure drop"
      mask help: Selects the ticked values from the thermo hydraulic vector.
      mask init:
      | v=[];
      | if (f)
      |     v  = [1];
      | end
      | if (t)
      |     v  = [v 2];
      | end
      | if (m)
      |     v= [v 3];
      | end
      | if (p)
      |     v = [v 4];
      | end
      | if (id)
      |     v = [v 5];
      | end
      | if (mix)
      |     v = [v 6];
      | end
      | if (d)
      |     v = [v 7];
      | end
      | if (dpcon)
      |     v = [v 8];
      | end
      | if (dplin)
      |     v = [v 9];
      | end
      | if (dpqua)
      |     v = [v 10];
      | end
      mask Help: eval('man(''THV_select'')')
  display_weather : Subsystem  mask(Select weather data){pos=off, sun_beam=off, sun_dfu=off, rad=on, ta=off, ts=off, pre=off, rh=off, ci=off, p=off, ws=off, wd=off, col=off}
      mask prompts: pos "sunposition [zenith azimuth incidence] angles [degree]"; sun_beam "solar beam radiation on a normal surface [W/m²]"; sun_dfu "solar diffuse radiation on a horizontal surface [W/m²]"; rad "solar radiation on the surface [direct diffuse] [W/m²]"; ta "ambient temperature [degree centigrade]"; ts "sky temperature [degree centigrade]"; pre "precipitation [m/s]"; rh "relative humidity [percent]"; ci "cloud index [0=no cloud 1= covered]"; p "pressure [Pa]"; ws "wind speed [m/s]"; wd "wind direction (0°=north 270°=east) [degree]"; col "collector [incidence parallel_incidence perpendicular] [degree]"
      mask help: Selects the ticked weather data from the input weather data vector.
      mask init:
      | v=[];
      | if (pos)
      |     v  = [2 3 14];
      | end
      | if (sun_beam)
      |     v= [v 4];
      | end
      | if (sun_dfu)
      |     v= [v 5];
      | end
      | if (rad)
      |     v= [v 17 18];
      | end
      | if (ta)
      |     v = [v 6];
      | end
      | if (ts)
      |     v = [v 7];
      | end
      | if (rh)
      |     v = [v 8];
      | end
      | if (pre)
      |     v = [v 9];
      | end
      | if (ci)
      |     v = [v 10];
      | end
      | if (p)
      |     v = [v 11];
      | end
      | if (ws)
      |     v = [v 12];
      | end
      | if (wd)
      |     v = [v 13];
      | end
      | if (col)
      |     v = [v 14 15 16];
      | end
      mask Help: web(fullfile(path_carnot('help'),'display_weather.html'),'-helpbrowser')
  printer : S-Function  FunctionName=printer  EnableBusSupport=off  mask(printer){}
      mask help: Print the input to the MATLAB command window during iterations of SIMULINK
      mask Help: web(fullfile(path_carnot('help'),'printer.html'),'-helpbrowser')
